simulink model "LoFT_Example3"  (R2024b)
settings: Solver=ode4  StartTime=0.0  StopTime=300  FixedStep=simu.dt  RelTol=1e-3
undefined symbols (not defined in the file): body, circtime, Communication, D1, Delta, irkb, line, LoFT, p0, Pn, s, simu, trip_time, Turbwind, waves, wind
libraries: simulink x350, spsThreePhaseVIMeasurementLib x41, spsThreePhasePISectionLineLib x34, spsThreePhaseParallelRLCLoadLib x21, spsThreePhaseTransformerTwoWindingsLib x14, spsLoadFlowBusLib x10, spsThreePhaseDynamicLoadLib x9, spsSynchronousMachinepuStandardLib x7, spsExcitationSystemLib x7, spsSteamTurbineandGovernorLib x7, spsGenericPowerSystemStabilizerLib x7, spsMultiBandPowerSystemStabilizerLib x7
(part 25 of 49)

== system LoFT_Example3/Onshore grid/Onshore Grid/Subsystem/SG6 ==
  Bus Selector1 : BusSelector  OutputSignals="Output active power   Peo (pu)"
  Bus Selector8 : BusSelector  OutputSignals="Output active power   Peo (pu),Output reactive power  Qeo (pu),Mechanical.Rotor speed  wm  (pu)"
  G6 : spsSynchronousMachinepuStandardLib/Synchronous Machine pu Standard  PresetModel=No  MechanicalLoad=Mechanical power Pm  ShowDetailedParameters=on  RotorType=Salient-pole  Units=per unit standard parameters  MeasurementBus=off  NominalParameters="[Pn(6,1)*1E9  22000   50 ]"  Reactances1=[ 31 32 33 34 35 36 37 ]  Reactances2=[ 1.305, 0.296, 0.252, 0.474, 0.243, 0.18 ]  dAxisTimeConstants=Short-circuit  qAxisTimeConstants=Open-circuit  TimeConstants1=[]  TimeConstants2=[]  TimeConstants3=[]  TimeConstants4=[]  TimeConstants5=[ 1.01, 0.053, 0.1 ]  TimeConstants6=[]  TimeConstants7=[]  TimeConstants8=[]  StatorResistance=2.8544e-3  Mechanical="[ 4.1 0  32]"  PolePairs=32  InitialConditions=[0 -74.7414 0.844209 0.844209 0.844209 -11.3603 -131.36 108.64 1.43001]  SetSaturation=off  Saturation=[0.6404,0.7127,0.8441,0.9214,0.9956,1.082,1.19,1.316,1.457;0.7,0.7698,0.8872,0.9466,0.9969,1.046,1.1,1.151,1.201]  LoadFlowParameters=[2 2133820000 0 0 0]  TsPowergui=0  TsBlock=-1  IterativeModel=Trapezoidal non iterative  IterativeDiscreteModel=Trapezoidal non iterative  BusType=PV  Pref=p0(6,1)*1E9  Qref=0  Qmin=-Inf  Qmax=Inf  PLF=0  QLF=0
  Regulators6 : Subsystem
  Scope13 : Scope  NumInputPorts=4
  A : PMIOPort  Side=Right
  B : PMIOPort  Port=2  Side=Right
  C : PMIOPort  Port=3  Side=Right
  tag scope: P_SG6=global
  wires:
  Bus Selector8/3 -> Scope13/3  "<Rotor speed  wm  (pu)>"
  Bus Selector8/2 -> Scope13/2  "<Output reactive power  Qeo (pu)>"
  G6/1 -> Bus Selector1/1, Bus Selector8/1, Regulators6/1(m)
  Bus Selector8/1 -> Scope13/1  "<Output active power   Peo (pu)>"
  Regulators6/1(Pm) -> G6/1
  Bus Selector1/1 -> [P_SG6]  "<Output active power   Peo (pu)>"
  Regulators6/2(Vf) -> Scope13/4, G6/2
  connections:
  G6/RConn1 -- A/RConn1
  G6/RConn2 -- B/RConn1
  G6/RConn3 -- C/RConn1

== system LoFT_Example3/Onshore grid/Onshore Grid/Subsystem/SG8 ==
  Bus Selector1 : BusSelector  OutputSignals="Output active power   Peo (pu)"
  Bus Selector2 : BusSelector  OutputSignals="Output active power   Peo (pu),Output reactive power  Qeo (pu),Mechanical.Rotor speed  wm  (pu)"
  G8 : spsSynchronousMachinepuStandardLib/Synchronous Machine pu Standard  PresetModel=No  MechanicalLoad=Mechanical power Pm  ShowDetailedParameters=on  RotorType=Salient-pole  Units=per unit standard parameters  MeasurementBus=off  NominalParameters="[Pn(8,1)*1e9  22000   50 ]"  Reactances1=[ 31 32 33 34 35 36 37 ]  Reactances2=[ 1.305, 0.296, 0.252, 0.474, 0.243, 0.18 ]  dAxisTimeConstants=Short-circuit  qAxisTimeConstants=Open-circuit  TimeConstants1=[]  TimeConstants2=[]  TimeConstants3=[]  TimeConstants4=[]  TimeConstants5=[ 1.01, 0.053, 0.1 ]  TimeConstants6=[]  TimeConstants7=[]  TimeConstants8=[]  StatorResistance=2.8544e-3  Mechanical="[ 4.1 0  32]"  PolePairs=32  InitialConditions=[0 -74.7414 0.844209 0.844209 0.844209 -11.3603 -131.36 108.64 1.43001]  SetSaturation=off  Saturation=[0.6404,0.7127,0.8441,0.9214,0.9956,1.082,1.19,1.316,1.457;0.7,0.7698,0.8872,0.9466,0.9969,1.046,1.1,1.151,1.201]  LoadFlowParameters=[2 2133820000 0 0 0]  TsPowergui=0  TsBlock=-1  IterativeModel=Trapezoidal non iterative  IterativeDiscreteModel=Trapezoidal non iterative  BusType=PV  Pref=p0(8,1)*1E9  Qref=0  Qmin=-Inf  Qmax=Inf  PLF=0  QLF=0
  Regulators8 : Subsystem
  Scope7 : Scope  NumInputPorts=4
  A : PMIOPort  Side=Right
  B : PMIOPort  Port=2  Side=Right
  C : PMIOPort  Port=3  Side=Right
  tag scope: P_SG8=global
  wires:
  Regulators8/2(Vf) -> Scope7/4, G8/2
  Bus Selector2/3 -> Scope7/3  "<Rotor speed  wm  (pu)>"
  Bus Selector2/2 -> Scope7/2  "<Output reactive power  Qeo (pu)>"
  Bus Selector2/1 -> Scope7/1  "<Output active power   Peo (pu)>"
  Regulators8/1(Pm) -> G8/1
  Bus Selector1/1 -> [P_SG8]  "<Output active power   Peo (pu)>"
  G8/1 -> Bus Selector1/1, Bus Selector2/1, Regulators8/1(m)
  connections:
  G8/RConn1 -- A/RConn1
  G8/RConn3 -- C/RConn1
  G8/RConn2 -- B/RConn1

== system LoFT_Example3/Onshore grid/Onshore Grid/Subsystem/SG9 ==
  Bus Selector1 : BusSelector  OutputSignals="Output active power   Peo (pu)"
  Bus Selector3 : BusSelector  OutputSignals="Output active power   Peo (pu),Output reactive power  Qeo (pu),Mechanical.Rotor speed  wm  (pu)"
  G9 : spsSynchronousMachinepuStandardLib/Synchronous Machine pu Standard  PresetModel=No  MechanicalLoad=Mechanical power Pm  ShowDetailedParameters=on  RotorType=Salient-pole  Units=per unit standard parameters  MeasurementBus=off  NominalParameters="[Pn(9,1)*1E9  22000   50 ]"  Reactances1=[ 31 32 33 34 35 36 37 ]  Reactances2=[ 1.305, 0.296, 0.252, 0.474, 0.243, 0.18 ]  dAxisTimeConstants=Short-circuit  qAxisTimeConstants=Open-circuit  TimeConstants1=[]  TimeConstants2=[]  TimeConstants3=[]  TimeConstants4=[]  TimeConstants5=[ 1.01, 0.053, 0.1 ]  TimeConstants6=[]  TimeConstants7=[]  TimeConstants8=[]  StatorResistance=2.8544e-3  Mechanical="[ 4.1 0  32]"  PolePairs=32  InitialConditions=[0 -74.7414 0.844209 0.844209 0.844209 -11.3603 -131.36 108.64 1.43001]  SetSaturation=off  Saturation=[0.6404,0.7127,0.8441,0.9214,0.9956,1.082,1.19,1.316,1.457;0.7,0.7698,0.8872,0.9466,0.9969,1.046,1.1,1.151,1.201]  LoadFlowParameters=[2 2133820000 0 0 0]  TsPowergui=0  TsBlock=-1  IterativeModel=Trapezoidal non iterative  IterativeDiscreteModel=Trapezoidal non iterative  BusType=PV  Pref=p0(9,1)*1E9  Qref=0  Qmin=-Inf  Qmax=Inf  PLF=0  QLF=0
  Regulators9 : Subsystem
  Scope8 : Scope  NumInputPorts=4
  A : PMIOPort  Side=Right
  B : PMIOPort  Port=2  Side=Right
  C : PMIOPort  Port=3  Side=Right
  tag scope: P_SG9=global
  wires:
  Regulators9/1(Pm) -> G9/1
  Regulators9/2(Vf) -> Scope8/4, G9/2
  Bus Selector3/2 -> Scope8/2  "<Output reactive power  Qeo (pu)>"
  Bus Selector3/3 -> Scope8/3  "<Rotor speed  wm  (pu)>"
  Bus Selector3/1 -> Scope8/1  "<Output active power   Peo (pu)>"
  Bus Selector1/1 -> [P_SG9]  "<Output active power   Peo (pu)>"
  G9/1 -> Bus Selector1/1, Bus Selector3/1, Regulators9/1(m)
  connections:
  C/RConn1 -- G9/RConn3
  B/RConn1 -- G9/RConn2
  A/RConn1 -- G9/RConn1

== system LoFT_Example3/Onshore grid/Onshore Grid/Subsystem/Subsystem1 ==
  In1 : Inport
  Constant : Constant
  Sum : Sum  Inputs=|++  SaturateOnIntegerOverflow=on
  tag scope: PSS_select=global
  wires:
  In1/1 -> Sum/1
  Sum/1 -> [PSS_select]
  Constant/1 -> Sum/2

== system LoFT_Example3/FOWT System/Subsystem1/FOWT1/Aerodynamics and Local Control Systems/Hull Aerodynamic ==
  In1 : Inport
  In2 : Inport  Port=2
  In4 : Inport  Port=3
  2-D Lookup Table1 : Lookup_n-D  BreakpointsForDimension1=Aero.TSR(1:1:24)  BreakpointsForDimension2=Aero.BlPitch(6:1:36)  Table=max(Aero.Ctmat(1:24,6:36),0)  InternalRulePriority=Speed  RndMeth=Simplest
      settings: InputPortMap=u0,u1
  Add1 : Sum
  Constant : Constant  Value=0
  Divide2 : Product  Inputs=*/
  Gain1 : Gain  Gain=0.5*1.225*pi*120^2*0.975*1.1
  Gain3 : Gain  Gain=120
  Gain5 : Gain  Gain=180/pi
  Product2 : Product
  Product3 : Product
  Saturation1 : Saturate  UpperLimit=2  LowerLimit=0
  Tower : Gain  Gain=0.613 * Aero.Cs * Aero.Ch * Aero.S
  Transfer Fcn2 : TransferFcn  Denominator=[0.2 1]
  Vector Concatenate1 : Concatenate  NumInputs=3
  mean force arm : Gain  Gain=92.8
  Out1 : Outport
  Rotor thrust : Outport  Port=2
  wires:
  Tower/1 -> Add1/1
  In1/1 -> Product2/2, Product2/1, Divide2/2
  Product3/1 -> Transfer Fcn2/1
  2-D Lookup Table1/1 -> Saturation1/1
  Saturation1/1 -> Gain1/1
  Add1/1 -> Rotor thrust/1, Vector Concatenate1/1, mean force arm/1
  Constant/1 -> Vector Concatenate1/2
  Transfer Fcn2/1 -> Add1/2
  Product2/1 -> Tower/1, Product3/1
  Divide2/1 -> 2-D Lookup Table1/1
  Gain3/1 -> Divide2/1
  Gain5/1 -> 2-D Lookup Table1/2
  Gain1/1 -> Product3/2
  mean force arm/1 -> Vector Concatenate1/3
  In2/1 -> Gain3/1
  In4/1 -> Gain5/1
  Vector Concatenate1/1 -> Out1/1

== system LoFT_Example3/FOWT System/Subsystem1/FOWT1/Aerodynamics and Local Control Systems/Local Control Systems ==
  WindSpeed : Inport
  RotSpeed : Inport  Port=2
  Nacelle Speed : Inport  Port=3
  " " : StateSpace  A=Controller.omegaFilter.A  B=Controller.omegaFilter.B  C=Controller.omegaFilter.C  D=Controller.omegaFilter.D  InitialCondition=[0,(7.55*pi/30)/Controller.omegaFilter.C(2)]
  Delay : Delay  DelayLength=1  InitialCondition=0
  Subsystem : Subsystem
  Subsystem1 : Subsystem
  Subsystem2 : Subsystem
  Transfer Fcn : TransferFcn  Denominator="[Controller.pitchFilter.A,   Controller.pitchFilter.B    1]"
  wind speed estimator : Subsystem
  GenTorq : Outport
  BldPitch : Outport  Port=2
  wires:
  WindSpeed/1 -> wind speed estimator/1(In1)
  " "/1 -> Subsystem/3(RotSpeed), Subsystem1/1(RotSpeed)
  Transfer Fcn/1 -> Subsystem1/4(Nacelle Speed)
  Nacelle Speed/1 -> Transfer Fcn/1
  RotSpeed/1 -> " "/1
  Subsystem2/1(Delta_omega_g) -> [Delta_omega_g]
  Subsystem1/1(BldPitch) -> BldPitch/1, Subsystem2/2(BldPitch)
  Subsystem/1(GenTorq) -> Subsystem2/1(GenTorq), GenTorq/1
  [Delta_omega_g] -> Delay/1
  Delay/1 -> Subsystem/2(2), Subsystem1/3(3)
  wind speed estimator/1(Out1) -> Subsystem/1(WindSpeed), Subsystem1/2(WindSpeed)

== system LoFT_Example3/FOWT System/Subsystem1/FOWT1/Aerodynamics and Local Control Systems/Rotor//drivetrain dynamics ==
  In1 : Inport
  In2 : Inport  Port=2
  In3 : Inport  Port=3
  In4 : Inport  Port=4
  In5 : Inport  Port=5
  1/J_rot : Gain  Gain=1/(LoFT.Property.rotorinertia)
  2-D Lookup Table : Lookup_n-D  BreakpointsForDimension1=Aero.TSR(1:1:24)  BreakpointsForDimension2=Aero.BlPitch(6:1:36)  Table=max(Aero.Cpmat(1:24,6:36),0)  InternalRulePriority=Speed  RndMeth=Simplest
      settings: InputPortMap=u0,u1
  Divide : Product  Inputs=**/
  Divide1 : Product  Inputs=*/
  Gain : Gain  Gain=0.5 * 1.225 * pi * 120^2 * 0.965 * 0.975
  Gain2 : Gain  Gain=120
  Gain4 : Gain  Gain=180/pi
  Integrator : Integrator  InitialCondition=Initstate(1)
  Product1 : Product  Inputs=3
  Saturation : Saturate  UpperLimit=1  LowerLimit=0
  Saturation3 : Saturate  UpperLimit=1.5  LowerLimit=0.3
  Sum : Sum  Inputs=|+-
  Transfer Fcn1 : TransferFcn  Denominator=[0.2 1]
  Out1 : Outport
  Out2 : Outport  Port=2
  wires:
  Saturation3/1 -> Out1/1, Divide/3
  Divide/1 -> Out2/1, Sum/1
  Divide1/1 -> 2-D Lookup Table/1
  Saturation/1 -> Gain/1
  In4/1 -> Product1/3, Product1/2, Product1/1
  Gain4/1 -> 2-D Lookup Table/2
  2-D Lookup Table/1 -> Saturation/1
  Transfer Fcn1/1 -> 1/J_rot/1
  In3/1 -> Gain4/1
  Integrator/1 -> Saturation3/1
  1/J_rot/1 -> Integrator/1
  Gain/1 -> Divide/1
  Gain2/1 -> Divide1/1
  Product1/1 -> Divide/2
  In5/1 -> Sum/2
  Sum/1 -> Transfer Fcn1/1
  In2/1 -> Divide1/2
  In1/1 -> Gain2/1

== system LoFT_Example3/FOWT System/Subsystem1/FOWT1/Aerodynamics and Local Control Systems/smooth1 ==
  In1 : Inport
  Gain : Gain  Gain=10
  Gain1 : Gain  Gain=10
  Integrator : Integrator  InitialCondition=0.1*8e6
  Scope : Scope  NumInputPorts=2
  Sum : Sum  Inputs=|+-
  Out1 : Outport
  wires:
  Gain1/1 -> Scope/2, Out1/1
  Integrator/1 -> Gain1/1, Gain/1
  Sum/1 -> Integrator/1
  Gain/1 -> Sum/2
  In1/1 -> Scope/1, Sum/1

== system LoFT_Example3/FOWT System/Subsystem1/FOWT1/Aerodynamics and Local Control Systems/wind speed estimator ==
  In1 : Inport
  Discrete Filter : DiscreteFilter  Numerator=Controller.F.Wind.b  Denominator=Controller.F.Wind.a  InitialStates=2000
  Out1 : Outport
  wires:
  In1/1 -> Discrete Filter/1
  Discrete Filter/1 -> Out1/1

== system LoFT_Example3/FOWT System/Subsystem1/FOWT1/Hydrodynamics/excitation force ==
  position : Inport
  Wave : Inport  Port=2
  Clock : Clock  Commented=on
  Frequency Spacing Delta Omega : Constant  Commented=on  Value=waves.dOmega/10  VectorParams1D=off
  Imaginary Part of Wave Excitation : Constant  Commented=on  Value=body.hydroForce.fExt.im(:,:,[1,3,5])  VectorParams1D=off
  Random Phase : Constant  Commented=on  Value=waves.phase  VectorParams1D=off
  Real Part of Wave Excitation : Constant  Commented=on  Value=body.hydroForce.fExt.re(:,:,[1,3,5])  VectorParams1D=off
  Real Part of Wave Excitation1 : Constant  Commented=on  Value=body.hydroForce.fExt.md(:,:,[1,3,5])  VectorParams1D=off
  WECSim Linear wave excitiation : MATLAB Function  Commented=on  TreatAsAtomicUnit=on
  Wave Frequency : Constant  Commented=on  Value=waves.omega/10  VectorParams1D=off
  Wave Spectrum : Constant  Commented=on  Value=waves.amplitude  VectorParams1D=off
  Wave direction spread : Constant  Commented=on  Value=waves.spread  VectorParams1D=off
  Wave direction1 : Constant  Commented=on  Value=waves.direction  VectorParams1D=off
  Fext : Outport
  wires:
  Wave/1 -> Fext/1
  Wave direction1/1 -> WECSim Linear wave excitiation/8(WaveDir)
  Frequency Spacing Delta Omega/1 -> WECSim Linear wave excitiation/6(dw)
  Wave Spectrum/1 -> WECSim Linear wave excitiation/1(A)
  Imaginary Part of Wave Excitation/1 -> WECSim Linear wave excitiation/4(fExtIM)
  Random Phase/1 -> WECSim Linear wave excitiation/5(phaseRand)
  Wave Frequency/1 -> WECSim Linear wave excitiation/2(w)
  Real Part of Wave Excitation1/1 -> WECSim Linear wave excitiation/10(fExtMD)
  Wave direction spread/1 -> WECSim Linear wave excitiation/9(spread)
  Clock/1 -> WECSim Linear wave excitiation/7(time)
  Real Part of Wave Excitation/1 -> WECSim Linear wave excitiation/3(fExtRE)

== system LoFT_Example3/FOWT System/Subsystem1/FOWT1/Hydrodynamics/radiation force ==
  velocity : Inport
  In2 : Inport  Port=2
  Add : Sum
  Constant1 : Constant  Value=Hydro.radiationaddedmass
  Constant2 : Constant  Value=Hydro.radiationdamping
  Demux : Demux  Commented=on  Outputs=3
  Demux1 : Demux  Commented=on  Outputs=3
  Gain : Gain  Commented=on  Gain=-1
  IRBK : Constant  Commented=on  Value=irkb(:,[1,3,5],[[1,3,5]])
  MATLAB Function : MATLAB Function  Commented=on  TreatAsAtomicUnit=on
  Product : Product  Multiplication=Matrix(*)
  Product1 : Product  Multiplication=Matrix(*)
  Rate Transition : RateTransition  Commented=on
  Reshape : Reshape  Commented=on
  Scope1 : Scope  Commented=on  NumInputPorts=2
  Scope2 : Scope  Commented=on  NumInputPorts=2
  Scope3 : Scope  Commented=on  NumInputPorts=2
  cicTime : Constant  Commented=on  Value=circtime
  F_rad : Outport
  wires:
  Add/1 -> F_rad/1
  Product/1 -> Add/1
  Constant2/1 -> Product1/1
  Constant1/1 -> Product/1
  In2/1 -> MATLAB Function/1(velocity), Product1/2
  IRBK/1 -> MATLAB Function/2(irkb)
  Rate Transition/1 -> Reshape/1
  cicTime/1 -> MATLAB Function/3(circtime)
  MATLAB Function/1(radiationdamping) -> Rate Transition/1
  velocity/1 -> Product/2
  Reshape/1 -> Gain/1
  Demux1/1 -> Scope1/1
  Demux/1 -> Scope1/2
  Demux1/2 -> Scope2/1
  Demux/2 -> Scope2/2
  Demux1/3 -> Scope3/1
  Demux/3 -> Scope3/2
  Gain/1 -> Demux/1
  Product1/1 -> Demux1/1, Add/2

== system LoFT_Example3/FOWT System/Subsystem1/FOWT1/Hydrodynamics/viscous force  ==
  In1 : Inport
  Abs : Abs  SaturateOnIntegerOverflow=off
  Constant3 : Constant  Value=Hydro.viscious
  Product2 : Product  Multiplication=Matrix(*)
  Product3 : Product
  F_vis : Outport
  wires:
  Product2/1 -> F_vis/1
  Product3/1 -> Product2/2
  In1/1 -> Product3/2, Abs/1
  Constant3/1 -> Product2/1
  Abs/1 -> Product3/1

== system LoFT_Example3/FOWT System/Subsystem1/FOWT1/wind speed(m//s)/smooth1 ==
  In1 : Inport
  Gain : Gain
  Gain1 : Gain
  Integrator : Integrator
  Scope : Scope  NumInputPorts=2
  Sum : Sum  Inputs=|+-
  FB : Outport
  wires:
  Gain1/1 -> Scope/2, FB/1
  Integrator/1 -> Gain1/1, Gain/1
  Sum/1 -> Integrator/1
  Gain/1 -> Sum/2
  In1/1 -> Scope/1, Sum/1

== system LoFT_Example3/FOWT System/Subsystem1/FOWT10/Aerodynamics and Local Control Systems/Hull Aerodynamic ==
  In1 : Inport
  In2 : Inport  Port=2
  In4 : Inport  Port=3
  2-D Lookup Table1 : Lookup_n-D  BreakpointsForDimension1=Aero.TSR(1:1:24)  BreakpointsForDimension2=Aero.BlPitch(6:1:36)  Table=max(Aero.Ctmat(1:24,6:36),0)  InternalRulePriority=Speed  RndMeth=Simplest
      settings: InputPortMap=u0,u1
  Add1 : Sum
  Constant : Constant  Value=0
  Divide2 : Product  Inputs=*/
  Gain1 : Gain  Gain=0.5*1.225*pi*120^2*0.975*1.1
  Gain3 : Gain  Gain=120
  Gain5 : Gain  Gain=180/pi
  Product2 : Product
  Product3 : Product
  Saturation1 : Saturate  UpperLimit=2  LowerLimit=0
  Tower : Gain  Gain=0.613 * Aero.Cs * Aero.Ch * Aero.S
  Transfer Fcn2 : TransferFcn  Denominator=[0.2 1]
  Vector Concatenate1 : Concatenate  NumInputs=3
  mean force arm : Gain  Gain=92.8
  Out1 : Outport
  Rotor thrust : Outport  Port=2
  wires:
  Vector Concatenate1/1 -> Out1/1
  In4/1 -> Gain5/1
  In2/1 -> Gain3/1
  mean force arm/1 -> Vector Concatenate1/3
  Gain1/1 -> Product3/2
  Gain5/1 -> 2-D Lookup Table1/2
  Gain3/1 -> Divide2/1
  Divide2/1 -> 2-D Lookup Table1/1
  Product2/1 -> Product3/1, Tower/1
  Transfer Fcn2/1 -> Add1/2
  Constant/1 -> Vector Concatenate1/2
  Add1/1 -> mean force arm/1, Vector Concatenate1/1, Rotor thrust/1
  Saturation1/1 -> Gain1/1
  2-D Lookup Table1/1 -> Saturation1/1
  Product3/1 -> Transfer Fcn2/1
  In1/1 -> Divide2/2, Product2/1, Product2/2
  Tower/1 -> Add1/1

== system LoFT_Example3/FOWT System/Subsystem1/FOWT10/Aerodynamics and Local Control Systems/Local Control Systems ==
  WindSpeed : Inport
  RotSpeed : Inport  Port=2
  Nacelle Speed : Inport  Port=3
  " " : StateSpace  A=Controller.omegaFilter.A  B=Controller.omegaFilter.B  C=Controller.omegaFilter.C  D=Controller.omegaFilter.D  InitialCondition=[0,(7.55*pi/30)/Controller.omegaFilter.C(2)]
  Delay : Delay  DelayLength=1  InitialCondition=0
  Subsystem : Subsystem
  Subsystem1 : Subsystem
  Subsystem2 : Subsystem
  Transfer Fcn : TransferFcn  Denominator="[Controller.pitchFilter.A,   Controller.pitchFilter.B    1]"
  wind speed estimator : Subsystem
  GenTorq : Outport
  BldPitch : Outport  Port=2
  wires:
  wind speed estimator/1(Out1) -> Subsystem1/2(WindSpeed), Subsystem/1(WindSpeed)
  Delay/1 -> Subsystem1/3(3), Subsystem/2(2)
  [Delta_omega_g] -> Delay/1
  Subsystem/1(GenTorq) -> GenTorq/1, Subsystem2/1(GenTorq)
  Subsystem1/1(BldPitch) -> Subsystem2/2(BldPitch), BldPitch/1
  Subsystem2/1(Delta_omega_g) -> [Delta_omega_g]
  RotSpeed/1 -> " "/1
  Nacelle Speed/1 -> Transfer Fcn/1
  Transfer Fcn/1 -> Subsystem1/4(Nacelle Speed)
  " "/1 -> Subsystem1/1(RotSpeed), Subsystem/3(RotSpeed)
  WindSpeed/1 -> wind speed estimator/1(In1)

== system LoFT_Example3/FOWT System/Subsystem1/FOWT10/Aerodynamics and Local Control Systems/Rotor//drivetrain dynamics ==
  In1 : Inport
  In2 : Inport  Port=2
  In3 : Inport  Port=3
  In4 : Inport  Port=4
  In5 : Inport  Port=5
  1/J_rot : Gain  Gain=1/(LoFT.Property.rotorinertia)
  2-D Lookup Table : Lookup_n-D  BreakpointsForDimension1=Aero.TSR(1:1:24)  BreakpointsForDimension2=Aero.BlPitch(6:1:36)  Table=max(Aero.Cpmat(1:24,6:36),0)  InternalRulePriority=Speed  RndMeth=Simplest
      settings: InputPortMap=u0,u1
  Divide : Product  Inputs=**/
  Divide1 : Product  Inputs=*/
  Gain : Gain  Gain=0.5 * 1.225 * pi * 120^2 * 0.965 * 0.975
  Gain2 : Gain  Gain=120
  Gain4 : Gain  Gain=180/pi
  Integrator : Integrator  InitialCondition=Initstate(1)
  Product1 : Product  Inputs=3
  Saturation : Saturate  UpperLimit=1  LowerLimit=0
  Saturation3 : Saturate  UpperLimit=1.5  LowerLimit=0.3
  Sum : Sum  Inputs=|+-
  Transfer Fcn1 : TransferFcn  Denominator=[0.2 1]
  Out1 : Outport
  Out2 : Outport  Port=2
  wires:
  In1/1 -> Gain2/1
  In2/1 -> Divide1/2
  Sum/1 -> Transfer Fcn1/1
  In5/1 -> Sum/2
  Product1/1 -> Divide/2
  Gain2/1 -> Divide1/1
  Gain/1 -> Divide/1
  1/J_rot/1 -> Integrator/1
  Integrator/1 -> Saturation3/1
  In3/1 -> Gain4/1
  Transfer Fcn1/1 -> 1/J_rot/1
  2-D Lookup Table/1 -> Saturation/1
  Gain4/1 -> 2-D Lookup Table/2
  In4/1 -> Product1/1, Product1/2, Product1/3
  Saturation/1 -> Gain/1
  Divide1/1 -> 2-D Lookup Table/1
  Divide/1 -> Sum/1, Out2/1
  Saturation3/1 -> Divide/3, Out1/1

== system LoFT_Example3/FOWT System/Subsystem1/FOWT10/Aerodynamics and Local Control Systems/smooth1 ==
  In1 : Inport
  Gain : Gain  Gain=10
  Gain1 : Gain  Gain=10
  Integrator : Integrator  InitialCondition=0.1*8e6
  Scope : Scope  NumInputPorts=2
  Sum : Sum  Inputs=|+-
  Out1 : Outport
  wires:
  In1/1 -> Sum/1, Scope/1
  Gain/1 -> Sum/2
  Sum/1 -> Integrator/1
  Integrator/1 -> Gain/1, Gain1/1
  Gain1/1 -> Out1/1, Scope/2

== system LoFT_Example3/FOWT System/Subsystem1/FOWT10/Aerodynamics and Local Control Systems/wind speed estimator ==
  In1 : Inport
  Discrete Filter : DiscreteFilter  Numerator=Controller.F.Wind.b  Denominator=Controller.F.Wind.a  InitialStates=2000
  Out1 : Outport
  wires:
  Discrete Filter/1 -> Out1/1
  In1/1 -> Discrete Filter/1

== system LoFT_Example3/FOWT System/Subsystem1/FOWT10/Hydrodynamics/excitation force ==
  position : Inport
  Wave : Inport  Port=2
  Clock : Clock  Commented=on
  Frequency Spacing Delta Omega : Constant  Commented=on  Value=waves.dOmega/10  VectorParams1D=off
  Imaginary Part of Wave Excitation : Constant  Commented=on  Value=body.hydroForce.fExt.im(:,:,[1,3,5])  VectorParams1D=off
  Random Phase : Constant  Commented=on  Value=waves.phase  VectorParams1D=off
  Real Part of Wave Excitation : Constant  Commented=on  Value=body.hydroForce.fExt.re(:,:,[1,3,5])  VectorParams1D=off
  Real Part of Wave Excitation1 : Constant  Commented=on  Value=body.hydroForce.fExt.md(:,:,[1,3,5])  VectorParams1D=off
  WECSim Linear wave excitiation : MATLAB Function  Commented=on  TreatAsAtomicUnit=on
  Wave Frequency : Constant  Commented=on  Value=waves.omega/10  VectorParams1D=off
  Wave Spectrum : Constant  Commented=on  Value=waves.amplitude  VectorParams1D=off
  Wave direction spread : Constant  Commented=on  Value=waves.spread  VectorParams1D=off
  Wave direction1 : Constant  Commented=on  Value=waves.direction  VectorParams1D=off
  Fext : Outport
  wires:
  Real Part of Wave Excitation/1 -> WECSim Linear wave excitiation/3(fExtRE)
  Clock/1 -> WECSim Linear wave excitiation/7(time)
  Wave direction spread/1 -> WECSim Linear wave excitiation/9(spread)
  Real Part of Wave Excitation1/1 -> WECSim Linear wave excitiation/10(fExtMD)
  Wave Frequency/1 -> WECSim Linear wave excitiation/2(w)
  Random Phase/1 -> WECSim Linear wave excitiation/5(phaseRand)
  Imaginary Part of Wave Excitation/1 -> WECSim Linear wave excitiation/4(fExtIM)
  Wave Spectrum/1 -> WECSim Linear wave excitiation/1(A)
  Frequency Spacing Delta Omega/1 -> WECSim Linear wave excitiation/6(dw)
  Wave direction1/1 -> WECSim Linear wave excitiation/8(WaveDir)
  Wave/1 -> Fext/1

== system LoFT_Example3/FOWT System/Subsystem1/FOWT10/Hydrodynamics/radiation force ==
  velocity : Inport
  In2 : Inport  Port=2
  Add : Sum
  Constant1 : Constant  Value=Hydro.radiationaddedmass
  Constant2 : Constant  Value=Hydro.radiationdamping
  Demux : Demux  Commented=on  Outputs=3
  Demux1 : Demux  Commented=on  Outputs=3
  Gain : Gain  Commented=on  Gain=-1
  IRBK : Constant  Commented=on  Value=irkb(:,[1,3,5],[[1,3,5]])
  MATLAB Function : MATLAB Function  Commented=on  TreatAsAtomicUnit=on
  Product : Product  Multiplication=Matrix(*)
  Product1 : Product  Multiplication=Matrix(*)
  Rate Transition : RateTransition  Commented=on
  Reshape : Reshape  Commented=on
  Scope1 : Scope  Commented=on  NumInputPorts=2
  Scope2 : Scope  Commented=on  NumInputPorts=2
  Scope3 : Scope  Commented=on  NumInputPorts=2
  cicTime : Constant  Commented=on  Value=circtime
  F_rad : Outport
  wires:
  Product1/1 -> Add/2, Demux1/1
  Gain/1 -> Demux/1
  Demux/3 -> Scope3/2
  Demux1/3 -> Scope3/1
  Demux/2 -> Scope2/2
  Demux1/2 -> Scope2/1
  Demux/1 -> Scope1/2
  Demux1/1 -> Scope1/1
  Reshape/1 -> Gain/1
  velocity/1 -> Product/2
  MATLAB Function/1(radiationdamping) -> Rate Transition/1
  cicTime/1 -> MATLAB Function/3(circtime)
  Rate Transition/1 -> Reshape/1
  IRBK/1 -> MATLAB Function/2(irkb)
  In2/1 -> Product1/2, MATLAB Function/1(velocity)
  Constant1/1 -> Product/1
  Constant2/1 -> Product1/1
  Product/1 -> Add/1
  Add/1 -> F_rad/1

== system LoFT_Example3/FOWT System/Subsystem1/FOWT10/Hydrodynamics/viscous force  ==
  In1 : Inport
  Abs : Abs  SaturateOnIntegerOverflow=off
  Constant3 : Constant  Value=Hydro.viscious
  Product2 : Product  Multiplication=Matrix(*)
  Product3 : Product
  F_vis : Outport
  wires:
  Abs/1 -> Product3/1
  Constant3/1 -> Product2/1
  In1/1 -> Abs/1, Product3/2
  Product3/1 -> Product2/2
  Product2/1 -> F_vis/1

== system LoFT_Example3/FOWT System/Subsystem1/FOWT10/wind speed(m//s)/smooth1 ==
  In1 : Inport
  Gain : Gain
  Gain1 : Gain
  Integrator : Integrator
  Scope : Scope  NumInputPorts=2
  Sum : Sum  Inputs=|+-
  FB : Outport
  wires:
  In1/1 -> Sum/1, Scope/1
  Gain/1 -> Sum/2
  Sum/1 -> Integrator/1
  Integrator/1 -> Gain/1, Gain1/1
  Gain1/1 -> FB/1, Scope/2

== system LoFT_Example3/FOWT System/Subsystem1/FOWT2/Aerodynamics and Local Control Systems/Hull Aerodynamic ==
  In1 : Inport
  In2 : Inport  Port=2
  In4 : Inport  Port=3
  2-D Lookup Table1 : Lookup_n-D  BreakpointsForDimension1=Aero.TSR(1:1:24)  BreakpointsForDimension2=Aero.BlPitch(6:1:36)  Table=max(Aero.Ctmat(1:24,6:36),0)  InternalRulePriority=Speed  RndMeth=Simplest
      settings: InputPortMap=u0,u1
  Add1 : Sum
  Constant : Constant  Value=0
  Divide2 : Product  Inputs=*/
  Gain1 : Gain  Gain=0.5*1.225*pi*120^2*0.975*1.1
  Gain3 : Gain  Gain=120
  Gain5 : Gain  Gain=180/pi
  Product2 : Product
  Product3 : Product
  Saturation1 : Saturate  UpperLimit=2  LowerLimit=0
  Tower : Gain  Gain=0.613 * Aero.Cs * Aero.Ch * Aero.S
  Transfer Fcn2 : TransferFcn  Denominator=[0.2 1]
  Vector Concatenate1 : Concatenate  NumInputs=3
  mean force arm : Gain  Gain=92.8
  Out1 : Outport
  Rotor thrust : Outport  Port=2
  wires:
  Vector Concatenate1/1 -> Out1/1
  In4/1 -> Gain5/1
  In2/1 -> Gain3/1
  mean force arm/1 -> Vector Concatenate1/3
  Gain1/1 -> Product3/2
  Gain5/1 -> 2-D Lookup Table1/2
  Gain3/1 -> Divide2/1
  Divide2/1 -> 2-D Lookup Table1/1
  Product2/1 -> Product3/1, Tower/1
  Transfer Fcn2/1 -> Add1/2
  Constant/1 -> Vector Concatenate1/2
  Add1/1 -> mean force arm/1, Vector Concatenate1/1, Rotor thrust/1
  Saturation1/1 -> Gain1/1
  2-D Lookup Table1/1 -> Saturation1/1
  Product3/1 -> Transfer Fcn2/1
  In1/1 -> Divide2/2, Product2/1, Product2/2
  Tower/1 -> Add1/1

== system LoFT_Example3/FOWT System/Subsystem1/FOWT2/Aerodynamics and Local Control Systems/Local Control Systems ==
  WindSpeed : Inport
  RotSpeed : Inport  Port=2
  Nacelle Speed : Inport  Port=3
  " " : StateSpace  A=Controller.omegaFilter.A  B=Controller.omegaFilter.B  C=Controller.omegaFilter.C  D=Controller.omegaFilter.D  InitialCondition=[0,(7.55*pi/30)/Controller.omegaFilter.C(2)]
  Delay : Delay  DelayLength=1  InitialCondition=0
  Subsystem : Subsystem
  Subsystem1 : Subsystem
  Subsystem2 : Subsystem
  Transfer Fcn : TransferFcn  Denominator="[Controller.pitchFilter.A,   Controller.pitchFilter.B    1]"
  wind speed estimator : Subsystem
  GenTorq : Outport
  BldPitch : Outport  Port=2
  wires:
  wind speed estimator/1(Out1) -> Subsystem1/2(WindSpeed), Subsystem/1(WindSpeed)
  Delay/1 -> Subsystem1/3(3), Subsystem/2(2)
  [Delta_omega_g] -> Delay/1
  Subsystem/1(GenTorq) -> GenTorq/1, Subsystem2/1(GenTorq)
  Subsystem1/1(BldPitch) -> Subsystem2/2(BldPitch), BldPitch/1
  Subsystem2/1(Delta_omega_g) -> [Delta_omega_g]
  RotSpeed/1 -> " "/1
  Nacelle Speed/1 -> Transfer Fcn/1
  Transfer Fcn/1 -> Subsystem1/4(Nacelle Speed)
  " "/1 -> Subsystem1/1(RotSpeed), Subsystem/3(RotSpeed)
  WindSpeed/1 -> wind speed estimator/1(In1)

== system LoFT_Example3/FOWT System/Subsystem1/FOWT2/Aerodynamics and Local Control Systems/Rotor//drivetrain dynamics ==
  In1 : Inport
  In2 : Inport  Port=2
  In3 : Inport  Port=3
  In4 : Inport  Port=4
  In5 : Inport  Port=5
  1/J_rot : Gain  Gain=1/(LoFT.Property.rotorinertia)
  2-D Lookup Table : Lookup_n-D  BreakpointsForDimension1=Aero.TSR(1:1:24)  BreakpointsForDimension2=Aero.BlPitch(6:1:36)  Table=max(Aero.Cpmat(1:24,6:36),0)  InternalRulePriority=Speed  RndMeth=Simplest
      settings: InputPortMap=u0,u1
  Divide : Product  Inputs=**/
  Divide1 : Product  Inputs=*/
  Gain : Gain  Gain=0.5 * 1.225 * pi * 120^2 * 0.965 * 0.975
  Gain2 : Gain  Gain=120
  Gain4 : Gain  Gain=180/pi
  Integrator : Integrator  InitialCondition=Initstate(1)
  Product1 : Product  Inputs=3
  Saturation : Saturate  UpperLimit=1  LowerLimit=0
  Saturation3 : Saturate  UpperLimit=1.5  LowerLimit=0.3
  Sum : Sum  Inputs=|+-
  Transfer Fcn1 : TransferFcn  Denominator=[0.2 1]
  Out1 : Outport
  Out2 : Outport  Port=2
  wires:
  In1/1 -> Gain2/1
  In2/1 -> Divide1/2
  Sum/1 -> Transfer Fcn1/1
  In5/1 -> Sum/2
  Product1/1 -> Divide/2
  Gain2/1 -> Divide1/1
  Gain/1 -> Divide/1
  1/J_rot/1 -> Integrator/1
  Integrator/1 -> Saturation3/1
  In3/1 -> Gain4/1
  Transfer Fcn1/1 -> 1/J_rot/1
  2-D Lookup Table/1 -> Saturation/1
  Gain4/1 -> 2-D Lookup Table/2
  In4/1 -> Product1/1, Product1/2, Product1/3
  Saturation/1 -> Gain/1
  Divide1/1 -> 2-D Lookup Table/1
  Divide/1 -> Sum/1, Out2/1
  Saturation3/1 -> Divide/3, Out1/1

== system LoFT_Example3/FOWT System/Subsystem1/FOWT2/Aerodynamics and Local Control Systems/smooth1 ==
  In1 : Inport
  Gain : Gain  Gain=10
  Gain1 : Gain  Gain=10
  Integrator : Integrator  InitialCondition=0.1*8e6
  Scope : Scope  NumInputPorts=2
  Sum : Sum  Inputs=|+-
  Out1 : Outport
  wires:
  In1/1 -> Sum/1, Scope/1
  Gain/1 -> Sum/2
  Sum/1 -> Integrator/1
  Integrator/1 -> Gain/1, Gain1/1
  Gain1/1 -> Out1/1, Scope/2

== system LoFT_Example3/FOWT System/Subsystem1/FOWT2/Aerodynamics and Local Control Systems/wind speed estimator ==
  In1 : Inport
  Discrete Filter : DiscreteFilter  Numerator=Controller.F.Wind.b  Denominator=Controller.F.Wind.a  InitialStates=2000
  Out1 : Outport
  wires:
  Discrete Filter/1 -> Out1/1
  In1/1 -> Discrete Filter/1

== system LoFT_Example3/FOWT System/Subsystem1/FOWT2/Hydrodynamics/excitation force ==
  position : Inport
  Wave : Inport  Port=2
  Clock : Clock  Commented=on
  Frequency Spacing Delta Omega : Constant  Commented=on  Value=waves.dOmega/10  VectorParams1D=off
  Imaginary Part of Wave Excitation : Constant  Commented=on  Value=body.hydroForce.fExt.im(:,:,[1,3,5])  VectorParams1D=off
  Random Phase : Constant  Commented=on  Value=waves.phase  VectorParams1D=off
  Real Part of Wave Excitation : Constant  Commented=on  Value=body.hydroForce.fExt.re(:,:,[1,3,5])  VectorParams1D=off
  Real Part of Wave Excitation1 : Constant  Commented=on  Value=body.hydroForce.fExt.md(:,:,[1,3,5])  VectorParams1D=off
  WECSim Linear wave excitiation : MATLAB Function  Commented=on  TreatAsAtomicUnit=on
  Wave Frequency : Constant  Commented=on  Value=waves.omega/10  VectorParams1D=off
  Wave Spectrum : Constant  Commented=on  Value=waves.amplitude  VectorParams1D=off
  Wave direction spread : Constant  Commented=on  Value=waves.spread  VectorParams1D=off
  Wave direction1 : Constant  Commented=on  Value=waves.direction  VectorParams1D=off
  Fext : Outport
  wires:
  Real Part of Wave Excitation/1 -> WECSim Linear wave excitiation/3(fExtRE)
  Clock/1 -> WECSim Linear wave excitiation/7(time)
  Wave direction spread/1 -> WECSim Linear wave excitiation/9(spread)
  Real Part of Wave Excitation1/1 -> WECSim Linear wave excitiation/10(fExtMD)
  Wave Frequency/1 -> WECSim Linear wave excitiation/2(w)
  Random Phase/1 -> WECSim Linear wave excitiation/5(phaseRand)
  Imaginary Part of Wave Excitation/1 -> WECSim Linear wave excitiation/4(fExtIM)
  Wave Spectrum/1 -> WECSim Linear wave excitiation/1(A)
  Frequency Spacing Delta Omega/1 -> WECSim Linear wave excitiation/6(dw)
  Wave direction1/1 -> WECSim Linear wave excitiation/8(WaveDir)
  Wave/1 -> Fext/1

== system LoFT_Example3/FOWT System/Subsystem1/FOWT2/Hydrodynamics/radiation force ==
  velocity : Inport
  In2 : Inport  Port=2
  Add : Sum
  Constant1 : Constant  Value=Hydro.radiationaddedmass
  Constant2 : Constant  Value=Hydro.radiationdamping
  Demux : Demux  Commented=on  Outputs=3
  Demux1 : Demux  Commented=on  Outputs=3
  Gain : Gain  Commented=on  Gain=-1
  IRBK : Constant  Commented=on  Value=irkb(:,[1,3,5],[[1,3,5]])
  MATLAB Function : MATLAB Function  Commented=on  TreatAsAtomicUnit=on
  Product : Product  Multiplication=Matrix(*)
  Product1 : Product  Multiplication=Matrix(*)
  Rate Transition : RateTransition  Commented=on
  Reshape : Reshape  Commented=on
  Scope1 : Scope  Commented=on  NumInputPorts=2
  Scope2 : Scope  Commented=on  NumInputPorts=2
  Scope3 : Scope  Commented=on  NumInputPorts=2
  cicTime : Constant  Commented=on  Value=circtime
  F_rad : Outport
  wires:
  Product1/1 -> Add/2, Demux1/1
  Gain/1 -> Demux/1
  Demux/3 -> Scope3/2
  Demux1/3 -> Scope3/1
  Demux/2 -> Scope2/2
  Demux1/2 -> Scope2/1
  Demux/1 -> Scope1/2
  Demux1/1 -> Scope1/1
  Reshape/1 -> Gain/1
  velocity/1 -> Product/2
  MATLAB Function/1(radiationdamping) -> Rate Transition/1
  cicTime/1 -> MATLAB Function/3(circtime)
  Rate Transition/1 -> Reshape/1
  IRBK/1 -> MATLAB Function/2(irkb)
  In2/1 -> Product1/2, MATLAB Function/1(velocity)
  Constant1/1 -> Product/1
  Constant2/1 -> Product1/1
  Product/1 -> Add/1
  Add/1 -> F_rad/1

== system LoFT_Example3/FOWT System/Subsystem1/FOWT2/Hydrodynamics/viscous force  ==
  In1 : Inport
  Abs : Abs  SaturateOnIntegerOverflow=off
  Constant3 : Constant  Value=Hydro.viscious
  Product2 : Product  Multiplication=Matrix(*)
  Product3 : Product
  F_vis : Outport
  wires:
  Abs/1 -> Product3/1
  Constant3/1 -> Product2/1
  In1/1 -> Abs/1, Product3/2
  Product3/1 -> Product2/2
  Product2/1 -> F_vis/1

== system LoFT_Example3/FOWT System/Subsystem1/FOWT2/wind speed(m//s)/smooth1 ==
  In1 : Inport
  Gain : Gain
  Gain1 : Gain
  Integrator : Integrator
  Scope : Scope  NumInputPorts=2
  Sum : Sum  Inputs=|+-
  FB : Outport
  wires:
  In1/1 -> Sum/1, Scope/1
  Gain/1 -> Sum/2
  Sum/1 -> Integrator/1
  Integrator/1 -> Gain/1, Gain1/1
  Gain1/1 -> FB/1, Scope/2

== system LoFT_Example3/FOWT System/Subsystem1/FOWT3/Aerodynamics and Local Control Systems/Hull Aerodynamic ==
  In1 : Inport
  In2 : Inport  Port=2
  In4 : Inport  Port=3
  2-D Lookup Table1 : Lookup_n-D  BreakpointsForDimension1=Aero.TSR(1:1:24)  BreakpointsForDimension2=Aero.BlPitch(6:1:36)  Table=max(Aero.Ctmat(1:24,6:36),0)  InternalRulePriority=Speed  RndMeth=Simplest
      settings: InputPortMap=u0,u1
  Add1 : Sum
  Constant : Constant  Value=0
  Divide2 : Product  Inputs=*/
  Gain1 : Gain  Gain=0.5*1.225*pi*120^2*0.975*1.1
  Gain3 : Gain  Gain=120
  Gain5 : Gain  Gain=180/pi
  Product2 : Product
  Product3 : Product
  Saturation1 : Saturate  UpperLimit=2  LowerLimit=0
  Tower : Gain  Gain=0.613 * Aero.Cs * Aero.Ch * Aero.S
  Transfer Fcn2 : TransferFcn  Denominator=[0.2 1]
  Vector Concatenate1 : Concatenate  NumInputs=3
  mean force arm : Gain  Gain=92.8
  Out1 : Outport
  Rotor thrust : Outport  Port=2
  wires:
  Tower/1 -> Add1/1
  In1/1 -> Product2/2, Product2/1, Divide2/2
  Product3/1 -> Transfer Fcn2/1
  2-D Lookup Table1/1 -> Saturation1/1
  Saturation1/1 -> Gain1/1
  Add1/1 -> Rotor thrust/1, Vector Concatenate1/1, mean force arm/1
  Constant/1 -> Vector Concatenate1/2
  Transfer Fcn2/1 -> Add1/2
  Product2/1 -> Tower/1, Product3/1
  Divide2/1 -> 2-D Lookup Table1/1
  Gain3/1 -> Divide2/1
  Gain5/1 -> 2-D Lookup Table1/2
  Gain1/1 -> Product3/2
  mean force arm/1 -> Vector Concatenate1/3
  In2/1 -> Gain3/1
  In4/1 -> Gain5/1
  Vector Concatenate1/1 -> Out1/1

== system LoFT_Example3/FOWT System/Subsystem1/FOWT3/Aerodynamics and Local Control Systems/Local Control Systems ==
  WindSpeed : Inport
  RotSpeed : Inport  Port=2
  Nacelle Speed : Inport  Port=3
  " " : StateSpace  A=Controller.omegaFilter.A  B=Controller.omegaFilter.B  C=Controller.omegaFilter.C  D=Controller.omegaFilter.D  InitialCondition=[0,(7.55*pi/30)/Controller.omegaFilter.C(2)]
  Delay : Delay  DelayLength=1  InitialCondition=0
  Subsystem : Subsystem
  Subsystem1 : Subsystem
  Subsystem2 : Subsystem
  Transfer Fcn : TransferFcn  Denominator="[Controller.pitchFilter.A,   Controller.pitchFilter.B    1]"
  wind speed estimator : Subsystem
  GenTorq : Outport
  BldPitch : Outport  Port=2
  wires:
  WindSpeed/1 -> wind speed estimator/1(In1)
  " "/1 -> Subsystem/3(RotSpeed), Subsystem1/1(RotSpeed)
  Transfer Fcn/1 -> Subsystem1/4(Nacelle Speed)
  Nacelle Speed/1 -> Transfer Fcn/1
  RotSpeed/1 -> " "/1
  Subsystem2/1(Delta_omega_g) -> [Delta_omega_g]
  Subsystem1/1(BldPitch) -> BldPitch/1, Subsystem2/2(BldPitch)
  Subsystem/1(GenTorq) -> Subsystem2/1(GenTorq), GenTorq/1
  [Delta_omega_g] -> Delay/1
  Delay/1 -> Subsystem/2(2), Subsystem1/3(3)
  wind speed estimator/1(Out1) -> Subsystem/1(WindSpeed), Subsystem1/2(WindSpeed)

== system LoFT_Example3/FOWT System/Subsystem1/FOWT3/Aerodynamics and Local Control Systems/Rotor//drivetrain dynamics ==
  In1 : Inport
  In2 : Inport  Port=2
  In3 : Inport  Port=3
  In4 : Inport  Port=4
  In5 : Inport  Port=5
  1/J_rot : Gain  Gain=1/(LoFT.Property.rotorinertia)
  2-D Lookup Table : Lookup_n-D  BreakpointsForDimension1=Aero.TSR(1:1:24)  BreakpointsForDimension2=Aero.BlPitch(6:1:36)  Table=max(Aero.Cpmat(1:24,6:36),0)  InternalRulePriority=Speed  RndMeth=Simplest
      settings: InputPortMap=u0,u1
  Divide : Product  Inputs=**/
  Divide1 : Product  Inputs=*/
  Gain : Gain  Gain=0.5 * 1.225 * pi * 120^2 * 0.965 * 0.975
  Gain2 : Gain  Gain=120
  Gain4 : Gain  Gain=180/pi
  Integrator : Integrator  InitialCondition=Initstate(1)
  Product1 : Product  Inputs=3
  Saturation : Saturate  UpperLimit=1  LowerLimit=0
  Saturation3 : Saturate  UpperLimit=1.5  LowerLimit=0.3
  Sum : Sum  Inputs=|+-
  Transfer Fcn1 : TransferFcn  Denominator=[0.2 1]
  Out1 : Outport
  Out2 : Outport  Port=2
  wires:
  Saturation3/1 -> Out1/1, Divide/3
  Divide/1 -> Out2/1, Sum/1
  Divide1/1 -> 2-D Lookup Table/1
  Saturation/1 -> Gain/1
  In4/1 -> Product1/3, Product1/2, Product1/1
  Gain4/1 -> 2-D Lookup Table/2
  2-D Lookup Table/1 -> Saturation/1
  Transfer Fcn1/1 -> 1/J_rot/1
  In3/1 -> Gain4/1
  Integrator/1 -> Saturation3/1
  1/J_rot/1 -> Integrator/1
  Gain/1 -> Divide/1
  Gain2/1 -> Divide1/1
  Product1/1 -> Divide/2
  In5/1 -> Sum/2
  Sum/1 -> Transfer Fcn1/1
  In2/1 -> Divide1/2
  In1/1 -> Gain2/1

== system LoFT_Example3/FOWT System/Subsystem1/FOWT3/Aerodynamics and Local Control Systems/smooth1 ==
  In1 : Inport
  Gain : Gain  Gain=10
  Gain1 : Gain  Gain=10
  Integrator : Integrator  InitialCondition=0.1*8e6
  Scope : Scope  NumInputPorts=2
  Sum : Sum  Inputs=|+-
  Out1 : Outport
  wires:
  Gain1/1 -> Scope/2, Out1/1
  Integrator/1 -> Gain1/1, Gain/1
  Sum/1 -> Integrator/1
  Gain/1 -> Sum/2
  In1/1 -> Scope/1, Sum/1

== system LoFT_Example3/FOWT System/Subsystem1/FOWT3/Aerodynamics and Local Control Systems/wind speed estimator ==
  In1 : Inport
  Discrete Filter : DiscreteFilter  Numerator=Controller.F.Wind.b  Denominator=Controller.F.Wind.a  InitialStates=2000
  Out1 : Outport
  wires:
  In1/1 -> Discrete Filter/1
  Discrete Filter/1 -> Out1/1

== system LoFT_Example3/FOWT System/Subsystem1/FOWT3/Hydrodynamics/excitation force ==
  position : Inport
  Wave : Inport  Port=2
  Clock : Clock  Commented=on
  Frequency Spacing Delta Omega : Constant  Commented=on  Value=waves.dOmega/10  VectorParams1D=off
  Imaginary Part of Wave Excitation : Constant  Commented=on  Value=body.hydroForce.fExt.im(:,:,[1,3,5])  VectorParams1D=off
  Random Phase : Constant  Commented=on  Value=waves.phase  VectorParams1D=off
  Real Part of Wave Excitation : Constant  Commented=on  Value=body.hydroForce.fExt.re(:,:,[1,3,5])  VectorParams1D=off
  Real Part of Wave Excitation1 : Constant  Commented=on  Value=body.hydroForce.fExt.md(:,:,[1,3,5])  VectorParams1D=off
  WECSim Linear wave excitiation : MATLAB Function  Commented=on  TreatAsAtomicUnit=on
  Wave Frequency : Constant  Commented=on  Value=waves.omega/10  VectorParams1D=off
  Wave Spectrum : Constant  Commented=on  Value=waves.amplitude  VectorParams1D=off
  Wave direction spread : Constant  Commented=on  Value=waves.spread  VectorParams1D=off
  Wave direction1 : Constant  Commented=on  Value=waves.direction  VectorParams1D=off
  Fext : Outport
  wires:
  Wave/1 -> Fext/1
  Wave direction1/1 -> WECSim Linear wave excitiation/8(WaveDir)
  Frequency Spacing Delta Omega/1 -> WECSim Linear wave excitiation/6(dw)
  Wave Spectrum/1 -> WECSim Linear wave excitiation/1(A)
  Imaginary Part of Wave Excitation/1 -> WECSim Linear wave excitiation/4(fExtIM)
  Random Phase/1 -> WECSim Linear wave excitiation/5(phaseRand)
  Wave Frequency/1 -> WECSim Linear wave excitiation/2(w)
  Real Part of Wave Excitation1/1 -> WECSim Linear wave excitiation/10(fExtMD)
  Wave direction spread/1 -> WECSim Linear wave excitiation/9(spread)
  Clock/1 -> WECSim Linear wave excitiation/7(time)
  Real Part of Wave Excitation/1 -> WECSim Linear wave excitiation/3(fExtRE)

== system LoFT_Example3/FOWT System/Subsystem1/FOWT3/Hydrodynamics/radiation force ==
  velocity : Inport
  In2 : Inport  Port=2
  Add : Sum
  Constant1 : Constant  Value=Hydro.radiationaddedmass
  Constant2 : Constant  Value=Hydro.radiationdamping
  Demux : Demux  Commented=on  Outputs=3
  Demux1 : Demux  Commented=on  Outputs=3
  Gain : Gain  Commented=on  Gain=-1
  IRBK : Constant  Commented=on  Value=irkb(:,[1,3,5],[[1,3,5]])
  MATLAB Function : MATLAB Function  Commented=on  TreatAsAtomicUnit=on
  Product : Product  Multiplication=Matrix(*)
  Product1 : Product  Multiplication=Matrix(*)
  Rate Transition : RateTransition  Commented=on
  Reshape : Reshape  Commented=on
  Scope1 : Scope  Commented=on  NumInputPorts=2
  Scope2 : Scope  Commented=on  NumInputPorts=2
  Scope3 : Scope  Commented=on  NumInputPorts=2
  cicTime : Constant  Commented=on  Value=circtime
  F_rad : Outport
  wires:
  Add/1 -> F_rad/1
  Product/1 -> Add/1
  Constant2/1 -> Product1/1
  Constant1/1 -> Product/1
  In2/1 -> MATLAB Function/1(velocity), Product1/2
  IRBK/1 -> MATLAB Function/2(irkb)
  Rate Transition/1 -> Reshape/1
  cicTime/1 -> MATLAB Function/3(circtime)
  MATLAB Function/1(radiationdamping) -> Rate Transition/1
  velocity/1 -> Product/2
  Reshape/1 -> Gain/1
  Demux1/1 -> Scope1/1
  Demux/1 -> Scope1/2
  Demux1/2 -> Scope2/1
  Demux/2 -> Scope2/2
  Demux1/3 -> Scope3/1
  Demux/3 -> Scope3/2
  Gain/1 -> Demux/1
  Product1/1 -> Demux1/1, Add/2

== system LoFT_Example3/FOWT System/Subsystem1/FOWT3/Hydrodynamics/viscous force  ==
  In1 : Inport
  Abs : Abs  SaturateOnIntegerOverflow=off
  Constant3 : Constant  Value=Hydro.viscious
  Product2 : Product  Multiplication=Matrix(*)
  Product3 : Product
  F_vis : Outport
  wires:
  Product2/1 -> F_vis/1
  Product3/1 -> Product2/2
  In1/1 -> Product3/2, Abs/1
  Constant3/1 -> Product2/1
  Abs/1 -> Product3/1

== system LoFT_Example3/FOWT System/Subsystem1/FOWT3/wind speed(m//s)/smooth1 ==
  In1 : Inport
  Gain : Gain
  Gain1 : Gain
  Integrator : Integrator
  Scope : Scope  NumInputPorts=2
  Sum : Sum  Inputs=|+-
  FB : Outport
  wires:
  Gain1/1 -> Scope/2, FB/1
  Integrator/1 -> Gain1/1, Gain/1
  Sum/1 -> Integrator/1
  Gain/1 -> Sum/2
  In1/1 -> Scope/1, Sum/1

== system LoFT_Example3/FOWT System/Subsystem1/FOWT4/Aerodynamics and Local Control Systems/Hull Aerodynamic ==
  In1 : Inport
  In2 : Inport  Port=2
  In4 : Inport  Port=3
  2-D Lookup Table1 : Lookup_n-D  BreakpointsForDimension1=Aero.TSR(1:1:24)  BreakpointsForDimension2=Aero.BlPitch(6:1:36)  Table=max(Aero.Ctmat(1:24,6:36),0)  InternalRulePriority=Speed  RndMeth=Simplest
      settings: InputPortMap=u0,u1
  Add1 : Sum
  Constant : Constant  Value=0
  Divide2 : Product  Inputs=*/
  Gain1 : Gain  Gain=0.5*1.225*pi*120^2*0.975*1.1
  Gain3 : Gain  Gain=120
  Gain5 : Gain  Gain=180/pi
  Product2 : Product
  Product3 : Product
  Saturation1 : Saturate  UpperLimit=2  LowerLimit=0
  Tower : Gain  Gain=0.613 * Aero.Cs * Aero.Ch * Aero.S
  Transfer Fcn2 : TransferFcn  Denominator=[0.2 1]
  Vector Concatenate1 : Concatenate  NumInputs=3
  mean force arm : Gain  Gain=92.8
  Out1 : Outport
  Rotor thrust : Outport  Port=2
  wires:
  Vector Concatenate1/1 -> Out1/1
  In4/1 -> Gain5/1
  In2/1 -> Gain3/1
  mean force arm/1 -> Vector Concatenate1/3
  Gain1/1 -> Product3/2
  Gain5/1 -> 2-D Lookup Table1/2
  Gain3/1 -> Divide2/1
  Divide2/1 -> 2-D Lookup Table1/1
  Product2/1 -> Product3/1, Tower/1
  Transfer Fcn2/1 -> Add1/2
  Constant/1 -> Vector Concatenate1/2
  Add1/1 -> mean force arm/1, Vector Concatenate1/1, Rotor thrust/1
  Saturation1/1 -> Gain1/1
  2-D Lookup Table1/1 -> Saturation1/1
  Product3/1 -> Transfer Fcn2/1
  In1/1 -> Divide2/2, Product2/1, Product2/2
  Tower/1 -> Add1/1

== system LoFT_Example3/FOWT System/Subsystem1/FOWT4/Aerodynamics and Local Control Systems/Local Control Systems ==
  WindSpeed : Inport
  RotSpeed : Inport  Port=2
  Nacelle Speed : Inport  Port=3
  " " : StateSpace  A=Controller.omegaFilter.A  B=Controller.omegaFilter.B  C=Controller.omegaFilter.C  D=Controller.omegaFilter.D  InitialCondition=[0,(7.55*pi/30)/Controller.omegaFilter.C(2)]
  Delay : Delay  DelayLength=1  InitialCondition=0
  Subsystem : Subsystem
  Subsystem1 : Subsystem
  Subsystem2 : Subsystem
  Transfer Fcn : TransferFcn  Denominator="[Controller.pitchFilter.A,   Controller.pitchFilter.B    1]"
  wind speed estimator : Subsystem
  GenTorq : Outport
  BldPitch : Outport  Port=2
  wires:
  wind speed estimator/1(Out1) -> Subsystem1/2(WindSpeed), Subsystem/1(WindSpeed)
  Delay/1 -> Subsystem1/3(3), Subsystem/2(2)
  [Delta_omega_g] -> Delay/1
  Subsystem/1(GenTorq) -> GenTorq/1, Subsystem2/1(GenTorq)
  Subsystem1/1(BldPitch) -> Subsystem2/2(BldPitch), BldPitch/1
  Subsystem2/1(Delta_omega_g) -> [Delta_omega_g]
  RotSpeed/1 -> " "/1
  Nacelle Speed/1 -> Transfer Fcn/1
  Transfer Fcn/1 -> Subsystem1/4(Nacelle Speed)
  " "/1 -> Subsystem1/1(RotSpeed), Subsystem/3(RotSpeed)
  WindSpeed/1 -> wind speed estimator/1(In1)

== system LoFT_Example3/FOWT System/Subsystem1/FOWT4/Aerodynamics and Local Control Systems/Rotor//drivetrain dynamics ==
  In1 : Inport
  In2 : Inport  Port=2
  In3 : Inport  Port=3
  In4 : Inport  Port=4
  In5 : Inport  Port=5
  1/J_rot : Gain  Gain=1/(LoFT.Property.rotorinertia)
  2-D Lookup Table : Lookup_n-D  BreakpointsForDimension1=Aero.TSR(1:1:24)  BreakpointsForDimension2=Aero.BlPitch(6:1:36)  Table=max(Aero.Cpmat(1:24,6:36),0)  InternalRulePriority=Speed  RndMeth=Simplest
      settings: InputPortMap=u0,u1
  Divide : Product  Inputs=**/
  Divide1 : Product  Inputs=*/
  Gain : Gain  Gain=0.5 * 1.225 * pi * 120^2 * 0.965 * 0.975
  Gain2 : Gain  Gain=120
  Gain4 : Gain  Gain=180/pi
  Integrator : Integrator  InitialCondition=Initstate(1)
  Product1 : Product  Inputs=3
  Saturation : Saturate  UpperLimit=1  LowerLimit=0
  Saturation3 : Saturate  UpperLimit=1.5  LowerLimit=0.3
  Sum : Sum  Inputs=|+-
  Transfer Fcn1 : TransferFcn  Denominator=[0.2 1]
  Out1 : Outport
  Out2 : Outport  Port=2
  wires:
  In1/1 -> Gain2/1
  In2/1 -> Divide1/2
  Sum/1 -> Transfer Fcn1/1
  In5/1 -> Sum/2
  Product1/1 -> Divide/2
  Gain2/1 -> Divide1/1
  Gain/1 -> Divide/1
  1/J_rot/1 -> Integrator/1
  Integrator/1 -> Saturation3/1
  In3/1 -> Gain4/1
  Transfer Fcn1/1 -> 1/J_rot/1
  2-D Lookup Table/1 -> Saturation/1
  Gain4/1 -> 2-D Lookup Table/2
  In4/1 -> Product1/1, Product1/2, Product1/3
  Saturation/1 -> Gain/1
  Divide1/1 -> 2-D Lookup Table/1
  Divide/1 -> Sum/1, Out2/1
  Saturation3/1 -> Divide/3, Out1/1

== system LoFT_Example3/FOWT System/Subsystem1/FOWT4/Aerodynamics and Local Control Systems/smooth1 ==
  In1 : Inport
  Gain : Gain  Gain=10
  Gain1 : Gain  Gain=10
  Integrator : Integrator  InitialCondition=0.1*8e6
  Scope : Scope  NumInputPorts=2
  Sum : Sum  Inputs=|+-
  Out1 : Outport
  wires:
  In1/1 -> Sum/1, Scope/1
  Gain/1 -> Sum/2
  Sum/1 -> Integrator/1
  Integrator/1 -> Gain/1, Gain1/1
  Gain1/1 -> Out1/1, Scope/2

== system LoFT_Example3/FOWT System/Subsystem1/FOWT4/Aerodynamics and Local Control Systems/wind speed estimator ==
  In1 : Inport
  Discrete Filter : DiscreteFilter  Numerator=Controller.F.Wind.b  Denominator=Controller.F.Wind.a  InitialStates=2000
  Out1 : Outport
  wires:
  Discrete Filter/1 -> Out1/1
  In1/1 -> Discrete Filter/1
